simulink model "cartPenSimModel"  (R2023b)
settings: Solver=VariableStepAuto  StartTime=0.0  StopTime=10.0  RelTol=1e-3
values from neighbouring files (symbols this model uses):
  Aa = [zeros(1,1) -C(2,:); zeros(4,1) A]    [e102finalproj.m]
  alpha = 0.5    [e102finalproj.m]
  Ba = [0; B]    [e102finalproj.m]
  Ca = [zeros(2,1) C]    [e102finalproj.m]
  Da = [D]    [e102finalproj.m]
  g = 9.8    [e102finalproj.m]
  K = augmentedK(2:5)    [e102finalproj.m]
  Ki = augmentedK(1)    [e102finalproj.m]
  L = place(Aa', Ca', obs_poles)    [e102finalproj.m]
libraries: cstblocks x1
settings Model: Creator=vparizot  LastModifiedBy=vparizot

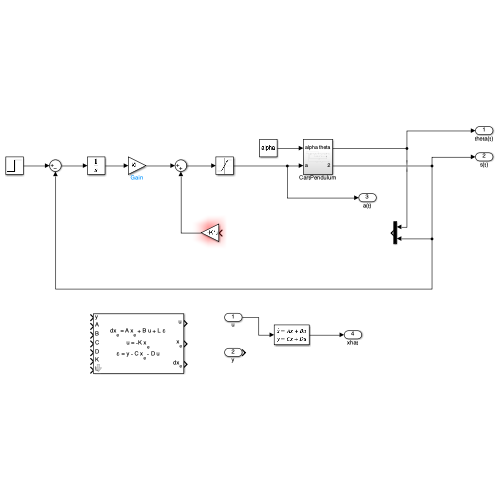
[thumbnail: Simulink's stored preview of the top-level diagram]
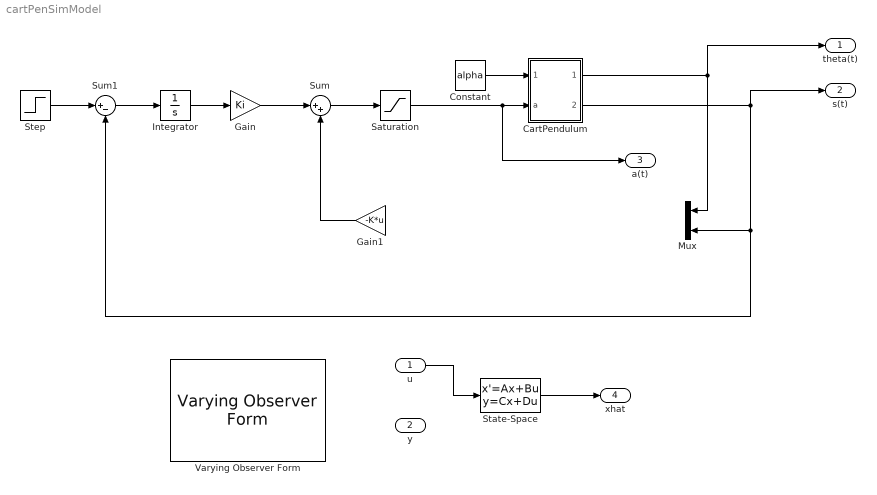
== system cartPenSimModel ==
  u : Inport
  y : Inport  Port=2
  CartPendulum : Subsystem
  Constant : Constant  Value=alpha
  Gain : Gain  Gain=Ki
  Gain1 : Gain  Gain=-K*u
  Integrator : Integrator
  Mux : Mux  Inputs=2
  Saturation : Saturate
  State-Space : StateSpace  A=Aa  B=Ba  C=Ca  D=Da  InitialCondition=0
  Step : Step  SampleTime=0
  Sum : Sum  Inputs=|++
  Sum1 : Sum  Inputs=|+-
  Varying Observer Form : cstblocks/Linear Parameter Varying/Varying Observer Form  x0=0  xNames=''  OutputX=on  OutputDX=on
  theta(t) : Outport
  s(t) : Outport  Port=2
  a(t) : Outport  Port=3
  xhat : Outport  Port=4
  wires:
  Integrator/1 -> Gain/1
  Gain/1 -> Sum/1
  Sum/1 -> Saturation/1
  Gain1/1 -> Sum/2
  Step/1 -> Sum1/1
  Sum1/1 -> Integrator/1
  Constant/1 -> CartPendulum/1(alpha)
  Saturation/1 -> a(t)/1, CartPendulum/2(a)
  CartPendulum/1(theta) -> theta(t)/1, Mux/1
  CartPendulum/2(Out2) -> s(t)/1, Sum1/2, Mux/2
  State-Space/1 -> xhat/1
  u/1 -> State-Space/1

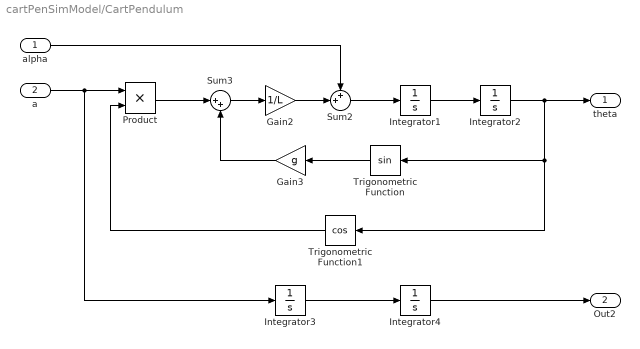
== system cartPenSimModel/CartPendulum ==
  alpha : Inport
  a : Inport  Port=2
  Gain2 : Gain  Gain=1/L
  Gain3 : Gain  Gain=g
  Integrator{1..4} (4 alike) : Integrator
  Product : Product
  Sum2 : Sum  Inputs=++|
  Sum3 : Sum  Inputs=|++
  Trigonometric Function : Trigonometry
  Trigonometric Function1 : Trigonometry  Operator=cos
  theta : Outport
  Out2 : Outport  Port=2
  wires:
  Trigonometric Function/1 -> Gain3/1
  alpha/1 -> Sum2/1
  Sum2/1 -> Integrator1/1
  Product/1 -> Sum3/1
  Integrator2/1 -> theta/1, Trigonometric Function/1, Trigonometric Function1/1
  Trigonometric Function1/1 -> Product/2
  Integrator1/1 -> Integrator2/1
  Integrator3/1 -> Integrator4/1
  Sum3/1 -> Gain2/1
  Integrator4/1 -> Out2/1
  Gain3/1 -> Sum3/2
  a/1 -> Product/1, Integrator3/1
  Gain2/1 -> Sum2/2
